simulink model "dop_rot_tb"  (R2016b)
settings: Solver=VariableStepAuto  StartTime=0.0  StopTime=10.0  RelTol=1e-3
undefined symbols (not defined in the file or in its folder): A, N
libraries: xbsIndex_r4 x18, simulink x5, dspbuff3 x4, dspswit3 x2, JTAGRuntimeCosim_r4 x1
settings Model: Creator=root  LastModifiedBy=root

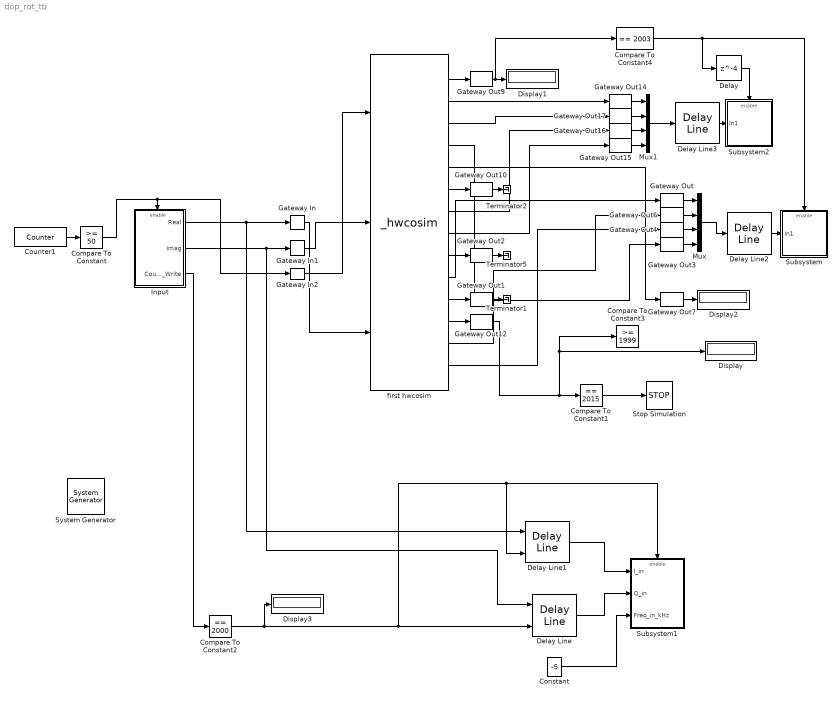
== system dop_rot_tb ==
  " System Generator" : xbsIndex_r4/ System Generator  Tag=genX  xilinxfamily=virtex7  part=xc7vx485t  speed=-2  package=ffg1761  synthesis_tool=Vivado  clock_wrapper=Clock Enables  directory=./netlist  proj_type=Vivado  Synth_file=Vivado Synthesis Defaults  Impl_file=Vivado Implementation Defaults  testbench=off  simulink_period=1/(70e6)  sysclk_period=1000/70  dcm_input_clock_period=10  incr_netlist=off  trim_vbits=Everywhere in SubSystem  dbl_ovrd=According to Block Masks  core_generation=According to Block Masks  run_coregen=off  deprecated_control=off  eval_field=0  block_type=sysgen
  Compare To Constant : simulink/Logic and Bit Operations/Compare To Constant  relop=>=  const=50  OutDataTypeStr=boolean
  Compare To Constant1 : simulink/Logic and Bit Operations/Compare To Constant  relop===  const=2015  OutDataTypeStr=boolean
  Compare To Constant2 : simulink/Logic and Bit Operations/Compare To Constant  relop===  const=2000  OutDataTypeStr=boolean
  Compare To Constant3 : simulink/Logic and Bit Operations/Compare To Constant  relop=>=  const=1999  OutDataTypeStr=boolean
  Compare To Constant4 : simulink/Logic and Bit Operations/Compare To Constant  relop===  const=2003  OutDataTypeStr=boolean
  Constant : Constant  Value=-5
  Counter1 : dspswit3/Counter  Direction=Up  CountEvent=Free running  CounterSize=16 bits  MaxCount=255  InitialCount=0  Output=Count  HitValue=32  ResetInput=off  SamplesPerFrame=1  Ts=1/(2e6)  CntDtype=uint16  HitDtype=Logical
  Delay : Delay  DelayLength=4  InitialCondition=0
  Delay Line : dspbuff3/Delay Line  siz=2000  ic=0  directfeed=on  enable_output=on  hold_output=on  TreatMby1Signals=One channel  OutputFrames=off
  Delay Line1 : dspbuff3/Delay Line  siz=2000  ic=0  directfeed=on  enable_output=on  hold_output=on  TreatMby1Signals=One channel  OutputFrames=off
  Delay Line2 : dspbuff3/Delay Line  siz=2000  ic=0  directfeed=on  enable_output=off  hold_output=on  TreatMby1Signals=One channel  OutputFrames=off
  Delay Line3 : dspbuff3/Delay Line  siz=2000  ic=0  directfeed=on  enable_output=off  hold_output=on  TreatMby1Signals=One channel  OutputFrames=off
  Display{,1..3} (4 alike) : Display
      settings: Format=decimal (Stored Integer)
  Gateway In : xbsIndex_r4/Gateway In  gui_display_data_type=Fixed-point  arith_type="Signed  (2's comp)"  n_bits=12  bin_pt=0  preci_type=Single  exp_width=8  frac_width=24  rows=1  columns=1  quantization="Round  (unbiased: +/- Inf)"  overflow=Saturate  period=1/(70e6)  UseAsADC=off  ADCChannel='1'  interface=None  automatic_assignment=on  address_offset=hex2dec('00')  intf_name=''  intf_description=''  default_value=0  timing_constraint=None  locs_specified=off  LOCs={}  io_standard={}  inherit_from_input=off  hdl_port=on  dbl_ovrd=off  block_type=gatewayin
  Gateway In1 : xbsIndex_r4/Gateway In  gui_display_data_type=Fixed-point  arith_type="Signed  (2's comp)"  n_bits=12  bin_pt=0  preci_type=Single  exp_width=8  frac_width=24  rows=1  columns=1  quantization="Round  (unbiased: +/- Inf)"  overflow=Saturate  period=1/(70e6)  UseAsADC=off  ADCChannel='1'  interface=None  automatic_assignment=on  address_offset=hex2dec('00')  intf_name=''  intf_description=''  default_value=0  timing_constraint=None  locs_specified=off  LOCs={}  io_standard={}  inherit_from_input=off  hdl_port=on  dbl_ovrd=off  block_type=gatewayin
  Gateway In2 : xbsIndex_r4/Gateway In  gui_display_data_type=Boolean  arith_type=Boolean  n_bits=16  bin_pt=0  preci_type=Single  exp_width=8  frac_width=24  rows=1  columns=1  quantization="Round  (unbiased: +/- Inf)"  overflow=Saturate  period=1/(2e6)  UseAsADC=off  ADCChannel='1'  interface=None  automatic_assignment=on  address_offset=hex2dec('00')  intf_name=''  intf_description=''  default_value=0  timing_constraint=None  locs_specified=off  LOCs={}  io_standard={}  inherit_from_input=off  hdl_port=on  dbl_ovrd=off  block_type=gatewayin
  Gateway Out{,1..4,6..7,9..10,12,14..17} (14 alike) : xbsIndex_r4/Gateway Out  inherit_from_input=on  hdl_port=on  rows=1  columns=1  UseAsDAC=off  DACChannel='1'  interface=None  automatic_assignment=on  address_offset=hex2dec('00')  intf_name=''  intf_description=''  timing_constraint=None  locs_specified=off  LOCs={}  io_standard={}  block_type=gatewayout
  "Input " : Subsystem
  Mux : Mux
  Mux1 : Mux
  Stop Simulation : Stop
  Subsystem : Subsystem
  Subsystem1 : Subsystem
  Subsystem2 : Subsystem
  Terminator1 : Terminator
  Terminator2 : Terminator
  Terminator5 : Terminator
  first hwcosim : JTAGRuntimeCosim_r4/_hwcosim  clkSrc=Single Stepped  hasCombinationalPath=on  bitfileName=/home/zaid/MTP/myrepo/sysgen/netlist/first.bit  skipConfig=off  dispPartInfo=off  useZynqReconfigScript=on  cable=Auto Detect  speed=N/A  cablePort=N/A  cableLocation=Local  shareCable=off  design_xtable=|  engineDll=JTAGCosimEngine.dll  cableWaitTime=10  bscanPos=-1  IRLengths=[]  useWaitBox=1  hasBufgmux=on  Scheme=Cosim  useCmdProc=1  hasProc=0  useImpact=0  printLogFile=0  userChain=2  block_type=jtagcosim
      | {
      |     'clkWrapper' => 'first',
      |     'burstMode' => false,
      |     'burstFifoDepth' => '1024',
      |     'shared_memories' => {},
      |     'clocksGcd' => 1,
      |     'device' => {
      |       'family' => 'virtex7',
      |       'part' => 'xc7vx485t',
      |       'package' => 'ffg1761',
      |       'speed' => '-2',
      |     },
      |     'ports' => {
      |       'gateway_in2' => {
      |         'direction' => 'in',
      |         'width' => 1,
      |         'name' => 'gateway_in2',
      |         'period' => 35,
      |         'icon_text' => 'Gateway In2',
      |         'type' => 'Bool',
      |         'arithmetic_type' => 'xlUnsigned',
      |         'dat_file' => 'first_gateway_in2.dat',
      |         'bin_pt' => 0,
      |         'addr_offset' => 0,
      |         'bd_port_index' => 0,
      |       },
      |       'gateway_in1' => {
      |         'direction' => 'in',
      |         'width' => 12,
      |         'name' => 'gateway_in1',
      |         'period' => 1,
      |         'icon_text' => 'Gateway In1',
      |         'type' => 'Fix_12_0',
      |         'arithmetic_type' => 'xlSigned',
      |         'dat_file' => 'first_gateway_in1.dat',
      |         'bin_pt' => 0,
      |         'addr_offset' => 4,
      |         'bd_port_index' => 1,
      |       },
      |       'gateway_in' => {
      |         'direction' => 'in',
      |         'width' => 12,
      |         'name' => 'gateway_in',
      |         'period' => 1,
      |         'icon_text' => 'Gateway In',
      |         'type' => 'Fix_12_0',
      |         'arithmetic_type' => 'xlSigned',
      |         'dat_file' => 'first_gateway_in.dat',
      |         'bin_pt' => 0,
      |         'addr_offset' => 8,
      |         'bd_port_index' => 2,
      |       },
      |       'gateway_out13' => {
      |         'direction' => 'out',
      |         'width' => 16,
      |         'name' => 'gateway_out13',
      |         'period' => 1,
      |         'icon_text' => 'Gateway Out13',
      |         'type' => 'UFix_16_0',
      |         'arithmetic_type' => 'xlUnsigned',
      |         'dat_file' => 'first_gateway_out13.dat',
      |         'bin_pt' => 0,
      |         'addr_offset' => 12,
      |         'bd_port_index' => 0,
      |       },
      |       'gateway_out' => {
      |         'direction' => 'out',
      |         'width' => 14,
      |         'name' => 'gateway_out',
      |         'period' => 1,
      |         'icon_text' => 'Gateway Out',
      |         'type' => 'UFix_14_0',
      |         'arithmetic_type' => 'xlUnsigned',
      |         'dat_file' => 'first_gateway_out.dat',
      |         'bin_pt' => 0,
      |         'addr_offset' => 16,
      |         'bd_port_index' => 1,
      |       },
      |       'gateway_out1' => {
      |         'direction' => 'out',
      |         'width' => 14,
      |         'name' => 'gateway_out1',
      |         'period' => 1,
      |         'icon_text' => 'Gateway Out1',
      |         'type' => 'UFix_14_0',
      |         'arithmetic_type' => 'xlUnsigned',
      |         'dat_file' => 'first_gateway_out1.dat',
      |         'bin_pt' => 0,
      |         'addr_offset' => 20,
      |         'bd_port_index' => 2,
      |       },
      |       'gateway_out10' => {
      |         'direction' => 'out',
      |         'width' => 12,
      |         'name' => 'gateway_out10',
      |         'period' => 1,
      |         'icon_text' => 'Gateway Out10',
      |         'type' => 'Fix_12_0',
      |         'arithmetic_type' => 'xlSigned',
      |         'dat_file' => 'first_gateway_out10.dat',
      |         'bin_pt' => 0,
      |         'addr_offset' => 24,
      |         'bd_port_index' => 3,
      |       },
      |       'gateway_out11' => {
      |         'direction' => 'out',
      |         'width' => 1,
      |         'name' => 'gateway_out11',
      |         'period' => 1,
      |         'icon_text' => 'Gateway Out11',
      |         'type' => 'UFix_1_0',
      |         'arithmetic_type' => 'xlUnsigned',
      |         'dat_file' => 'first_gateway_out11.dat',
      |         'bin_pt' => 0,
      |         'addr_offset' => 28,
      |         'bd_port_index' => 4,
      |       },
      |       'gateway_out12' => {
      |         'direction' => 'out',
      |         'width' => 1,
      |         'name' => 'gateway_out12',
      |         'period' => 1,
      |         'icon_text' => 'Gateway Out12',
      |         'type' => 'UFix_1_0',
      |         'arithmetic_type' => 'xlUnsigned',
      |         'dat_file' => 'first_gateway_out12.dat',
      |         'bin_pt' => 0,
      |         'addr_offset' => 32,
      |         'bd_port_index' => 5,
      |       },
      |       'gateway_out2' => {
      |         'direction' => 'out',
      |         'width' => 14,
      |         'name' => 'gateway_out2',
      |         'period' => 1,
      |         'icon_text' => 'Gateway Out2',
      |         'type' => 'UFix_14_0',
      |         'arithmetic_type' => 'xlUnsigned',
      |         'dat_file' => 'first_gateway_out2.dat',
      |         'bin_pt' => 0,
      |         'addr_offset' => 36,
      |         'bd_port_index' => 6,
      |       },
      |       'gateway_out3' => {
      |         'direction' => 'out',
      |         'width' => 14,
      |         'name' => 'gateway_out3',
      |         'period' => 1,
      |         'icon_text' => 'Gateway Out3',
      |         'type' => 'UFix_14_0',
      |         'arithmetic_type' => 'xlUnsigned',
      |         'dat_file' => 'first_gateway_out3.dat',
      |         'bin_pt' => 0,
      |         'addr_offset' => 40,
      |         'bd_port_index' => 7,
      |       },
      |       'gateway_out4' => {
      |         'direction' => 'out',
      |         'width' => 32,
      |         'name' => 'gateway_out4',
      |         'period' => 1,
      |         'icon_text' => 'Gateway Out4',
      |         'type' => 'UFix_32_0',
      |         'arithmetic_type' => 'xlUnsigned',
      |         'dat_file' => 'first_gateway_out4.dat',
      |         'bin_pt' => 0,
      |         'addr_offset' => 44,
      |         'bd_port_index' => 8,
      |       },
      |       'gateway_out5' => {
      |         'direction' => 'out',
      |         'width' => 12,
      |         'name' => 'gateway_out5',
      |         'period' => 1,
      |         'icon_text' => 'Gateway Out5',
      |         'type' => 'Fix_12_0',
      |         'arithmetic_type' => 'xlSigned',
      |         'dat_file' => 'first_gateway_out5.dat',
      |         'bin_pt' => 0,
      |         'addr_offset' => 48,
      |         'bd_port_index' => 9,
      |       },
      |       'gateway_out6' => {
      |         'direction' => 'out',
      |         'width' => 12,
      |         'name' => 'gateway_out6',
      |         'period' => 1,
      |         'icon_text' => 'Gateway Out6',
      |         'type' => 'Fix_12_0',
      |         'arithmetic_type' => 'xlSigned',
      |         'dat_file' => 'first_gateway_out6.dat',
      |         'bin_pt' => 0,
      |         'addr_offset' => 52,
      |         'bd_port_index' => 10,
      |       },
      |       'gateway_out7' => {
      |         'direction' => 'out',
      |         'width' => 16,
      |         'name' => 'gateway_out7',
      |         'period' => 35,
      |         'icon_text' => 'Gateway Out7',
      |         'type' => 'UFix_16_0',
      |         'arithmetic_type' => 'xlUnsigned',
      |         'dat_file' => 'first_gateway_out7.dat',
      |         'bin_pt' => 0,
      |         'addr_offset' => 56,
      |         'bd_port_index' => 11,
      |       },
      |       'gateway_out8' => {
      |         'direction' => 'out',
      |         'width' => 12,
      |         'name' => 'gateway_out8',
      |         'period' => 1,
      |         'icon_text' => 'Gateway Out8',
      |         'type' => 'Fix_12_0',
      |         'arithmetic_type' => 'xlSigned',
      |         'dat_file' => 'first_gateway_out8.dat',
      |         'bin_pt' => 0,
      |         'addr_offset' => 60,
      |         'bd_port_index' => 12,
      |       },
      |       'gateway_out9' => {
      |         'direction' => 'out',
      |         'width' => 12,
      |         'name' => 'gateway_out9',
      |         'period' => 1,
      |         'icon_text' => 'Gateway Out9',
      |         'type' => 'Fix_12_0',
      |         'arithmetic_type' => 'xlSigned',
      |         'dat_file' => 'first_gateway_out9.dat',
      |         'bin_pt' => 0,
      |         'addr_offset' => 64,
      |         'bd_port_index' => 13,
      |       },
      |     },
      |   }
  wires:
  "Input "/1(Real) -> Delay Line1/1, Gateway In/1
  Counter1/1 -> Compare To Constant/1
  Compare To Constant/1 -> Gateway In2/1, "Input "/Enable
  Gateway In2/1 -> first hwcosim/1
  first hwcosim/10 -> Gateway Out/1
  first hwcosim/4 -> Gateway Out3/1
  first hwcosim/14 -> Gateway Out4/1
  Gateway In/1 -> first hwcosim/3
  Gateway In1/1 -> first hwcosim/2
  first hwcosim/13 -> Gateway Out6/1
  first hwcosim/5 -> Gateway Out7/1
  "Input "/3("Count_Write ") -> Compare To Constant2/1
  Delay Line/1 -> Subsystem1/2(Q_in)
  "Input "/2("Imag ") -> Delay Line/1, Gateway In1/1
  Compare To Constant2/1 -> Display3/1, Subsystem1/Enable, Delay Line1/2, Delay Line/2
  Delay Line1/1 -> Subsystem1/1(I_in)
  Constant/1 -> Subsystem1/3("Freq_in_kHz ")
  Gateway Out/1 -> Mux/1
  Gateway Out6/1 -> Mux/2
  Gateway Out4/1 -> Mux/3
  Gateway Out3/1 -> Mux/4
  Mux/1 -> Delay Line2/1
  first hwcosim/12 -> Gateway Out12/1
  Gateway Out12/1 -> Compare To Constant3/1, Display/1, Compare To Constant1/1
  first hwcosim/11 -> Gateway Out1/1
  first hwcosim/9 -> Gateway Out2/1
  first hwcosim/1 -> Gateway Out9/1
  first hwcosim/6 -> Gateway Out10/1
  Gateway Out1/1 -> Terminator1/1
  Gateway Out10/1 -> Terminator2/1
  first hwcosim/7 -> Gateway Out16/1
  first hwcosim/8 -> Gateway Out15/1
  Gateway Out2/1 -> Terminator5/1
  first hwcosim/3 -> Gateway Out17/1
  first hwcosim/2 -> Gateway Out14/1
  Delay Line2/1 -> Subsystem/1(In1)
  Gateway Out7/1 -> Display2/1
  Gateway Out9/1 -> Compare To Constant4/1, Display1/1
  Compare To Constant1/1 -> Stop Simulation/1
  Gateway Out14/1 -> Mux1/1
  Gateway Out17/1 -> Mux1/2
  Gateway Out16/1 -> Mux1/3
  Gateway Out15/1 -> Mux1/4
  Mux1/1 -> Delay Line3/1
  Compare To Constant4/1 -> Delay/1, Subsystem/Enable
  Delay Line3/1 -> Subsystem2/1(In1)
  Delay/1 -> Subsystem2/Enable

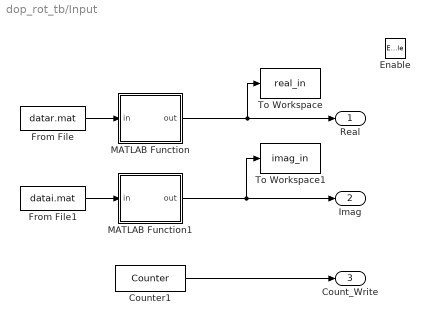
== system dop_rot_tb/Input  ==
  Enable : EnablePort
  Counter1 : dspswit3/Counter  Direction=Up  CountEvent=Free running  CounterSize=User defined  MaxCount=2000  InitialCount=1  Output=Count  HitValue=32  ResetInput=off  SamplesPerFrame=1  Ts=1/(2e6)  CntDtype=uint16  HitDtype=Logical
  From File : FromFile  FileName=datar.mat  SampleTime=1/(2e6)
  From File1 : FromFile  FileName=datai.mat  SampleTime=1/(2e6)
  MATLAB Function : MATLAB Function  TreatAsAtomicUnit=on
  MATLAB Function1 : MATLAB Function  TreatAsAtomicUnit=on
  To Workspace : ToWorkspace  VariableName=real_in  SaveFormat=Timeseries  SampleTime=-1
  To Workspace1 : ToWorkspace  VariableName=imag_in  SaveFormat=Timeseries  SampleTime=-1
  Real : Outport
  "Imag " : Outport  Port=2
  "Count_Write " : Outport  Port=3
  wires:
  From File1/1 -> MATLAB Function1/1(in)
  MATLAB Function/1(out) -> To Workspace/1, Real/1
  From File/1 -> MATLAB Function/1(in)
  MATLAB Function1/1(out) -> To Workspace1/1, "Imag "/1
  Counter1/1 -> "Count_Write "/1

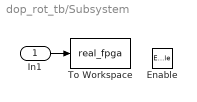
== system dop_rot_tb/Subsystem ==
  In1 : Inport
  Enable : EnablePort
  To Workspace : ToWorkspace  VariableName=real_fpga  SaveFormat=Timeseries  SampleTime=-1
  wires:
  In1/1 -> To Workspace/1

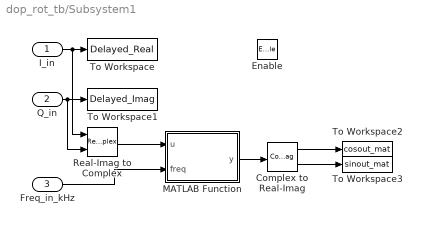
== system dop_rot_tb/Subsystem1 ==
  I_in : Inport
  Q_in : Inport  Port=2
  "Freq_in_kHz " : Inport  Port=3
  Enable : EnablePort
  Complex to Real-Imag : ComplexToRealImag
  MATLAB Function : MATLAB Function  TreatAsAtomicUnit=on
  Real-Imag to Complex : RealImagToComplex
  To Workspace : ToWorkspace  VariableName=Delayed_Real  SaveFormat=Timeseries  SampleTime=-1
  To Workspace1 : ToWorkspace  VariableName=Delayed_Imag  SaveFormat=Timeseries  SampleTime=-1
  To Workspace2 : ToWorkspace  VariableName=cosout_mat  SaveFormat=Timeseries  SampleTime=-1
  To Workspace3 : ToWorkspace  VariableName=sinout_mat  SaveFormat=Timeseries  SampleTime=-1
  wires:
  I_in/1 -> Real-Imag to Complex/1, To Workspace/1
  Q_in/1 -> Real-Imag to Complex/2, To Workspace1/1
  Real-Imag to Complex/1 -> MATLAB Function/1(u)
  "Freq_in_kHz "/1 -> MATLAB Function/2(freq)
  MATLAB Function/1(y) -> Complex to Real-Imag/1
  Complex to Real-Imag/1 -> To Workspace2/1
  Complex to Real-Imag/2 -> To Workspace3/1

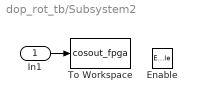
== system dop_rot_tb/Subsystem2 ==
  In1 : Inport
  Enable : EnablePort
  To Workspace : ToWorkspace  VariableName=cosout_fpga  SaveFormat=Timeseries  SampleTime=-1
  wires:
  In1/1 -> To Workspace/1

== matlab function dop_rot_tb/Input /MATLAB Function1 ==
  data: in input; out output
function out=toint(in)
in=in*2^16;
in=round(in);
out=fix(in);

== matlab function dop_rot_tb/Input /MATLAB Function ==
  data: in input; out output
function out=toint(in)
in=in*2^16;
in=round(in);
out=fix(in);

== matlab function dop_rot_tb/Subsystem1/MATLAB Function ==
  data: u input; freq input; y output
function y=fcn(u,freq)
sample_time=1/(2e6);
time_axis=0:sample_time:sample_time*(length(u)-1);
carrier=exp(1i*2*pi*freq*time_axis*1e3);
y = u.*(carrier.');
y=fix(round(y*cordic_scale(16)));
